simulink model "HumpbackBridgeSubBlock"  (R2018b)
settings: Solver=ode45  StartTime=0.0  StopTime=10.0  MaxStep=0.01  RelTol=1e-3  EnableMultiTasking=on
settings Model: Creator=acookson  LastModifiedBy=Reece Bell
settings DataIOCC: LimitDataPoints=on  SaveFormat=Array
settings OptimizationCC: LifeSpan=inf
settings DebuggingCC: SolverPrmCheckMsg=warning  SFUnexpectedBacktrackingDiag=warning  SFNoUnconditionalDefaultTransitionDiag=warning  SFExecutionAtInitializationDiag=none
settings HardwareCC: ProdBitPerPointer=32  ProdBitPerSizeT=32  ProdBitPerPtrDiffT=32  ProdLargestAtomicFloat=None  ProdIntDivRoundTo=Undefined  ProdEndianess=Unspecified  ProdWordSize=32  ProdHWDeviceType=32-bit Generic
settings ModelReferenceCC: PropagateSignalLabelsOutOfModel=off
settings SFSimCC: SimUseLocalCustomCode=off
settings RTWCC: RTWUseLocalCustomCode=off
settings CodeAppCC: StateflowObjectComments=on
settings GRTTargetCC: TargetLangStandard=C89/C90 (ANSI)  GeneratePreprocessorConditionals=Disable all
settings ConfigComp: CovMetricSettings=dw  CovHtmlReporting=on  CovSaveCumulativeToWorkspaceVar=on  CovSaveSingleToWorkspaceVar=on  CovExternalEMLEnable=off  CovSFcnEnable=off

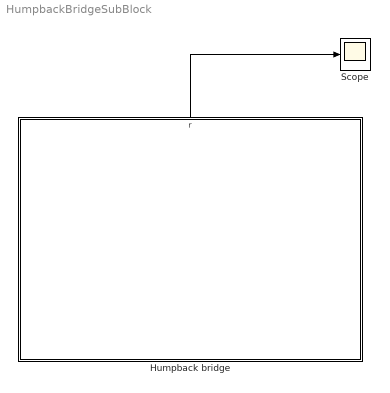
== system HumpbackBridgeSubBlock ==
  Humpback bridge : Subsystem  mask{h=2, L=20, v=20}
      mask prompts: h "humpback height (m)"; L "humpback length (m)"; v "vehicle speed (m/s)"
  Scope : Scope
  wires:
  Humpback bridge/1(r) -> Scope/1

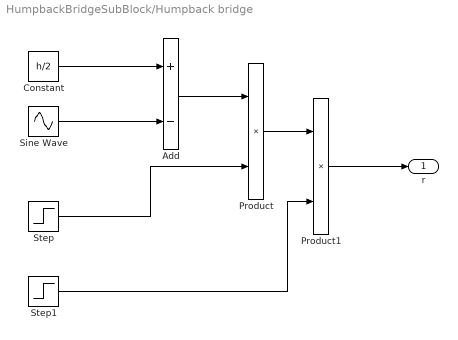
== system HumpbackBridgeSubBlock/Humpback bridge ==
  Add : Sum  Inputs=+-
  Constant : Constant  Value=h/2
  Product : Product
  Product1 : Product
  Sine Wave : Sin  Amplitude=h/2  Frequency=2*pi*v/L  Phase=pi/2  SampleTime=0
  Step : Step  Time=2*L/v  SampleTime=0
  Step1 : Step  Time=3*L/v  Before=1  After=0  SampleTime=0
  r : Outport
  wires:
  Constant/1 -> Add/1
  Sine Wave/1 -> Add/2
  Add/1 -> Product/1
  Step/1 -> Product/2
  Product/1 -> Product1/1
  Step1/1 -> Product1/2
  Product1/1 -> r/1
